simulink model "adaptive"  (R2018a)
settings: Solver=FixedStepAuto  StartTime=0.0  StopTime=20  FixedStep=Ts  RelTol=1e-3
values from neighbouring files (symbols this model uses):
  gammaa = 5    [parameter.m]
  gammap = 2    [parameter.m]
  lamdaa = 5    [parameter.m]
  lamdap = 3    [parameter.m]
  rhop = 2    [parameter.m]
settings Model: Creator=DuyNam  LastModifiedBy=DuyNam

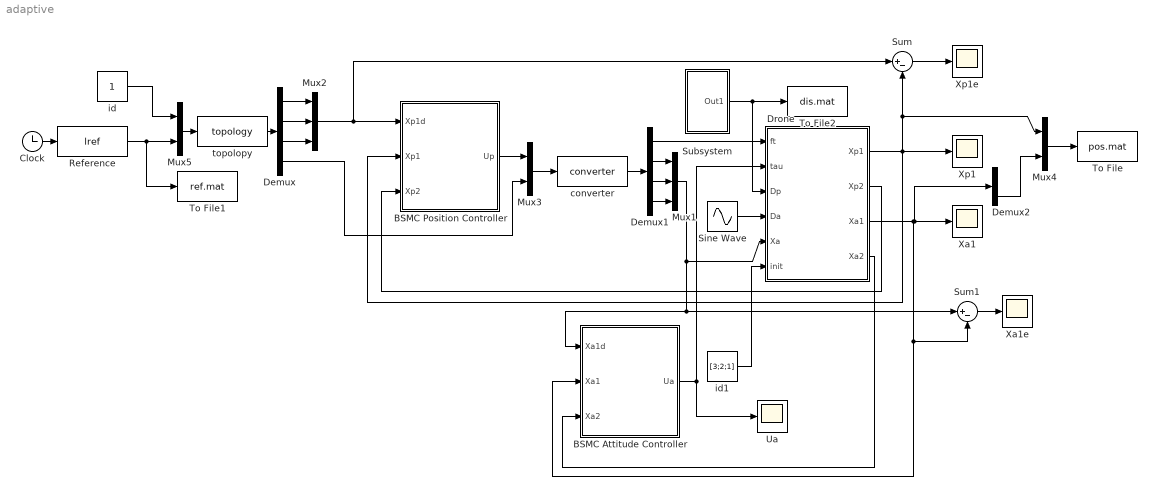
== system adaptive ==
  BSMC Attitude Controller : Subsystem
  BSMC Position Controller : Subsystem
  Clock : Clock
  Demux : Demux
  Demux1 : Demux
  Demux2 : Demux  Outputs=3
  Drone : Subsystem
  Mux1 : Mux  Inputs=3
  Mux2 : Mux  Inputs=3
  Mux3 : Mux  Inputs=2
  Mux4 : Mux  Inputs=2
  Mux5 : Mux  Inputs=2
  Reference : MATLABFcn  MATLABFcn=lref  OutputDimensions=4
  Sine Wave : Sin  Amplitude=[0;0;0]  Frequency=2*pi/10  SampleTime=0
  Subsystem : Subsystem
  Sum : Sum  Inputs=|+-
  Sum1 : Sum  Inputs=|+-
  To File : ToFile  Filename=pos.mat  SaveFormat=Timeseries
  To File1 : ToFile  Filename=ref.mat  SaveFormat=Timeseries
  To File2 : ToFile  Filename=dis.mat  SaveFormat=Timeseries
  Ua : Scope
  Xa1 : Scope
  Xa1e : Scope
  Xp1 : Scope
  Xp1e : Scope
  converter : MATLABFcn  MATLABFcn=converter  OutputDimensions=4
  id : Constant
  id1 : Constant  Value=[3;2;1]
  "topolopy " : MATLABFcn  MATLABFcn=topology  OutputDimensions=4
  wires:
  Sum/1 -> Xp1e/1
  Reference/1 -> To File1/1, Mux5/2
  Demux/1 -> Mux2/1
  Demux/2 -> Mux2/2
  Demux/3 -> Mux2/3
  Mux2/1 -> Sum/1, BSMC Position Controller/1(Xp1d)
  Demux/4 -> Mux3/2
  Mux3/1 -> converter/1
  BSMC Position Controller/1(Up) -> Mux3/1
  Clock/1 -> Reference/1
  converter/1 -> Demux1/1
  Demux1/3 -> Mux1/2
  Demux1/2 -> Mux1/1
  Demux1/4 -> Mux1/3
  Mux1/1 -> Drone/5(Xa), Sum1/1, BSMC Attitude Controller/1(Xa1d)
  Sum1/1 -> Xa1e/1
  Drone/1(Xp1) -> Mux4/1, Sum/2, Xp1/1, BSMC Position Controller/2(Xp1)
  Drone/3(Xa1) -> Demux2/1, Xa1/1, BSMC Attitude Controller/2(Xa1), Sum1/2
  Demux1/1 -> Drone/1(ft)
  BSMC Attitude Controller/1(Ua) -> Ua/1, Drone/2(tau)
  Drone/2(Xp2) -> BSMC Position Controller/3(Xp2)
  Drone/4(Xa2) -> BSMC Attitude Controller/3(Xa2)
  Sine Wave/1 -> Drone/4(Da)
  Subsystem/1(Out1) -> To File2/1, Drone/3(Dp)
  Mux4/1 -> To File/1
  Demux2/3 -> Mux4/2
  "topolopy "/1 -> Demux/1
  Mux5/1 -> "topolopy "/1
  id/1 -> Mux5/1
  id1/1 -> Drone/6(init)

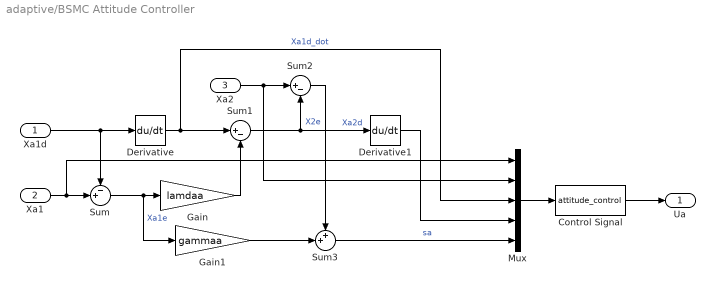
== system adaptive/BSMC Attitude Controller ==
  Xa1d : Inport
  Xa1 : Inport  Port=2
  Xa2 : Inport  Port=3
  Control Signal : MATLABFcn  MATLABFcn=attitude_control  OutputDimensions=3
  Derivative : Derivative
  Derivative1 : Derivative
  Gain : Gain  Gain=lamdaa
  Gain1 : Gain  Gain=gammaa
  Mux : Mux  Inputs=5
  Sum : Sum  Inputs=-+|
  Sum1 : Sum  Inputs=|+-
  Sum2 : Sum  Inputs=|+-
  Sum3 : Sum  Inputs=++|
  Ua : Outport
  wires:
  Xa1d/1 -> Sum/1, Derivative/1
  Xa1/1 -> Mux/1, Sum/2
  Sum/1 -> Gain1/1, Gain/1  "Xa1e"
  Derivative/1 -> Sum1/1, Mux/3  "Xa1d_dot"
  Gain/1 -> Sum1/2
  Sum1/1 -> Derivative1/1, Sum2/2  "Xa2d"
  Xa2/1 -> Mux/2, Sum2/1
  Sum2/1 -> Sum3/1  "X2e"
  Gain1/1 -> Sum3/2
  Sum3/1 -> Mux/5  "sa"
  Mux/1 -> Control Signal/1
  Derivative1/1 -> Mux/4
  Control Signal/1 -> Ua/1

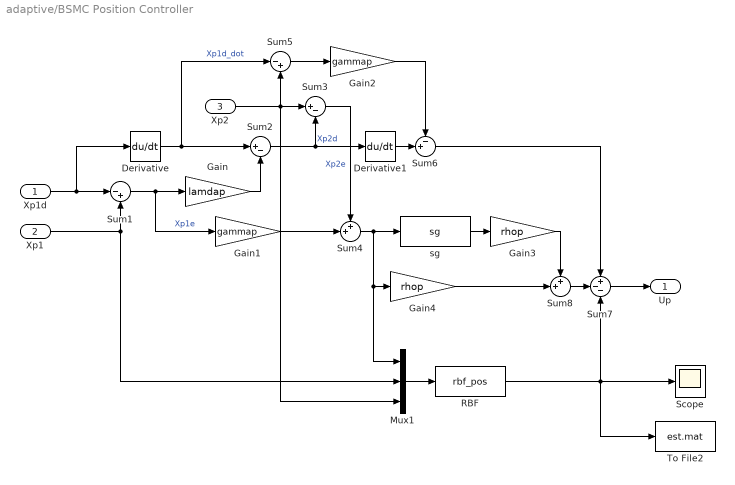
== system adaptive/BSMC Position Controller ==
  Xp1d : Inport
  Xp1 : Inport  Port=2
  Xp2 : Inport  Port=3
  Derivative : Derivative
  Derivative1 : Derivative
  Gain : Gain  Gain=lamdap
  Gain1 : Gain  Gain=gammap
  Gain2 : Gain  Gain=gammap
  Gain3 : Gain  Gain=rhop
  Gain4 : Gain  Gain=rhop
  Mux1 : Mux  Inputs=3
  RBF : MATLABFcn  MATLABFcn=rbf_pos  OutputDimensions=3
  Scope : Scope
  Sum1 : Sum  Inputs=|-+
  Sum2 : Sum  Inputs=|+-
  Sum3 : Sum  Inputs=|+-
  Sum4 : Sum  Inputs=++|
  Sum5 : Sum  Inputs=|-+
  Sum6 : Sum  Inputs=-+|
  Sum7 : Sum  Inputs=+--
  Sum8 : Sum  Inputs=++|
  To File2 : ToFile  Filename=est.mat  SaveFormat=Timeseries
  sg : MATLABFcn  MATLABFcn=sg
  Up : Outport
  wires:
  Xp1d/1 -> Derivative/1, Sum1/1
  Sum1/1 -> Gain1/1, Gain/1  "Xp1e"
  Derivative/1 -> Sum5/1, Sum2/1  "Xp1d_dot"
  Gain/1 -> Sum2/2
  Sum2/1 -> Derivative1/1, Sum3/2  "Xp2d"
  Sum3/1 -> Sum4/1  "Xp2e"
  Gain1/1 -> Sum4/2
  Sum5/1 -> Gain2/1
  Derivative1/1 -> Sum6/2
  Gain2/1 -> Sum6/1
  sg/1 -> Gain3/1
  Sum6/1 -> Sum7/1
  Sum7/1 -> Up/1
  Gain3/1 -> Sum8/1
  Gain4/1 -> Sum8/2
  Sum8/1 -> Sum7/2
  RBF/1 -> Sum7/3, To File2/1, Scope/1
  Xp2/1 -> Sum5/2, Sum3/1, Mux1/3
  Sum4/1 -> sg/1, Mux1/1, Gain4/1
  Mux1/1 -> RBF/1
  Xp1/1 -> Mux1/2, Sum1/2

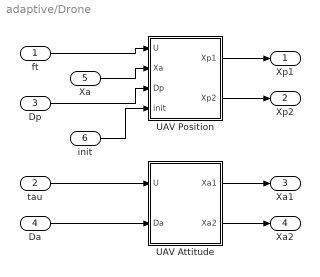
== system adaptive/Drone ==
  ft : Inport
  tau : Inport  Port=2
  Dp : Inport  Port=3
  Da : Inport  Port=4
  Xa : Inport  Port=5
  init : Inport  Port=6
  UAV Attitude : Subsystem
  UAV Position : Subsystem
  Xp1 : Outport
  Xp2 : Outport  Port=2
  Xa1 : Outport  Port=3
  Xa2 : Outport  Port=4
  wires:
  UAV Attitude/2(Xa2) -> Xa2/1
  tau/1 -> UAV Attitude/1(U)
  UAV Position/1(Xp1) -> Xp1/1
  UAV Position/2(Xp2) -> Xp2/1
  ft/1 -> UAV Position/1(U)
  Dp/1 -> UAV Position/3(Dp)
  Da/1 -> UAV Attitude/2(Da)
  UAV Attitude/1(Xa1) -> Xa1/1
  Xa/1 -> UAV Position/2(Xa)
  init/1 -> UAV Position/4("init ")

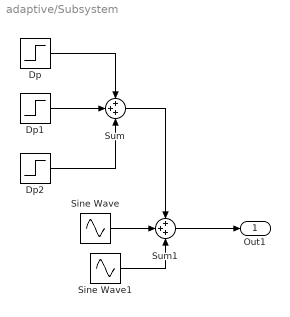
== system adaptive/Subsystem ==
  Dp : Step  Time=5  After=[10;15;5]  SampleTime=0
  Dp1 : Step  Time=10  After=[5;-5;6]  SampleTime=0
  Dp2 : Step  Time=15  After=[-4;-9;-5]  SampleTime=0
  Sine Wave : Sin  Amplitude=[4,-3,3]  Frequency=pi/3  SampleTime=0
  Sine Wave1 : Sin  Amplitude=[-3,2,1]  Frequency=2*pi/3  SampleTime=0
  Sum : Sum  Inputs=+++
  Sum1 : Sum  Inputs=+++
  Out1 : Outport
  wires:
  Dp/1 -> Sum/1
  Dp1/1 -> Sum/2
  Dp2/1 -> Sum/3
  Sum1/1 -> Out1/1
  Sum/1 -> Sum1/1
  Sine Wave/1 -> Sum1/2
  Sine Wave1/1 -> Sum1/3

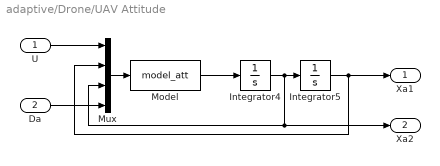
== system adaptive/Drone/UAV Attitude ==
  U : Inport
  Da : Inport  Port=2
  Integrator4 : Integrator
  Integrator5 : Integrator
  Model : MATLABFcn  MATLABFcn=model_att  OutputDimensions=3
  Mux : Mux
  Xa1 : Outport
  Xa2 : Outport  Port=2
  wires:
  Integrator5/1 -> Mux/2, Xa1/1
  Mux/1 -> Model/1
  U/1 -> Mux/1
  Model/1 -> Integrator4/1
  Integrator4/1 -> Integrator5/1, Xa2/1, Mux/3
  Da/1 -> Mux/4

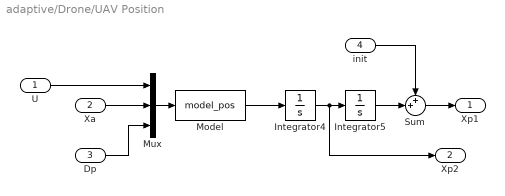
== system adaptive/Drone/UAV Position ==
  U : Inport
  Xa : Inport  Port=2
  Dp : Inport  Port=3
  "init " : Inport  Port=4
  Integrator4 : Integrator
  Integrator5 : Integrator
  Model : MATLABFcn  MATLABFcn=model_pos  OutputDimensions=3
  Mux : Mux  Inputs=3
  Sum : Sum  Inputs=++|
  Xp1 : Outport
  Xp2 : Outport  Port=2
  wires:
  Integrator4/1 -> Xp2/1, Integrator5/1
  Integrator5/1 -> Sum/2
  Model/1 -> Integrator4/1
  U/1 -> Mux/1
  Mux/1 -> Model/1
  Xa/1 -> Mux/2
  Dp/1 -> Mux/3
  Sum/1 -> Xp1/1
  "init "/1 -> Sum/1
